simulink model "Praktikum05"  (R2023b)
settings: Solver=VariableStepAuto  StartTime=0.0  StopTime=0.01  RelTol=1e-3
model workspace (MAT data in the model file):
  CodeRate = 0.75
  M = 16
  PunctureVector = [1; 1; 0; 1; 0; 1]
  TracebackDepth = 48
  Trelli.numInputSymbols = 2
  Trelli.numOutputSymbols = 4
  Trelli.numStates = 64
  Trelli.nextStates = [0  32; 0  32; 1  33; 1  33; 2  34; 2  34; 3  35; 3  35; 4  36; 4  36; 5  37; 5  37; 6  38; 6  38; 7  39; 7  39; 8  40; 8  40; 9  41; 9  41; 10  42; 10  42; 11  43; 11  43; 12  44; 12  44; 13  45; 13  45; 14  46; 14  46; 15  47; 15  47; 16  48; 16  48; 17  49; 17  49; 18  50; 18  50; 19  51; 19  51; 20  52; 20  52; 21  53; 21  53; 22  54; 22  54; 23  55; 23  55; 24  56; 24  56; 25  57; 25  57; 26  58; 26  58; 27  59; 27  59; 28  60; 28  60; 29  61; 29  61; 30  62; 30  62; 31  63; 31  63]
  Trelli.outputs = [0  3; 3  0; 1  2; 2  1; 0  3; 3  0; 1  2; 2  1; 3  0; 0  3; 2  1; 1  2; 3  0; 0  3; 2  1; 1  2; 3  0; 0  3; 2  1; 1  2; 3  0; 0  3; 2  1; 1  2; 0  3; 3  0; 1  2; 2  1; 0  3; 3  0; 1  2; 2  1; 2  1; 1  2; 3  0; 0  3; 2  1; 1  2; 3  0; 0  3; 1  2; 2  1; 0  3; 3  0; 1  2; 2  1; 0  3; 3  0; 1  2; 2  1; 0  3; 3  0; 1  2; 2  1; 0  3; 3  0; 2  1; 1  2; 3  0; 0  3; 2  1; 1  2; 3  0; 0  3]
  Ts = 5e-08
undefined symbols (not defined in the file or in its folder): doppler, magnitude
libraries: commchan3 x2, commrflib2 x2, commsink2 x2, commdigbbndam3 x2, dspquant2 x2, commcnvcod2 x2, dspxfrm3 x1, dspstat3 x1, dspindex x1, dspmathops x1
settings Model: Creator=suttarar@hu-berlin.de  LastModifiedBy=suttarar@hu-berlin.de

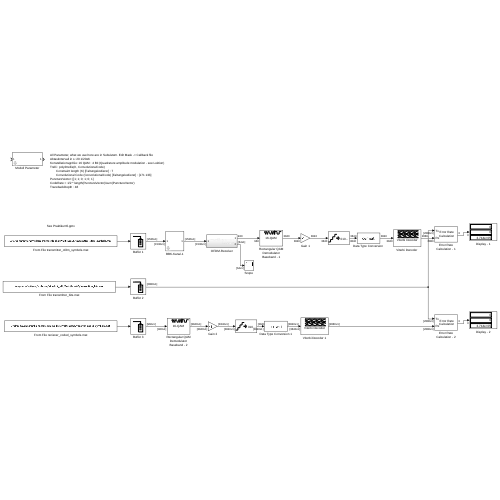
[thumbnail: Simulink's stored preview of the top-level diagram]
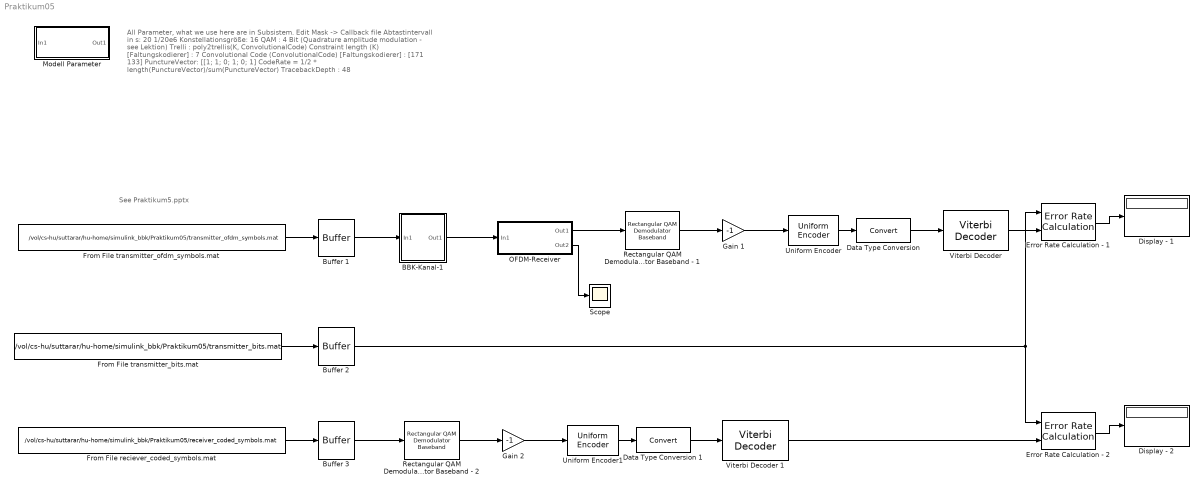
== system Praktikum05 ==
  note: See Praktikum5.pptx
  note: All Parameter, what we use here are in Subsistem. Edit Mask -> Callback file
      | Abtastintervall in s: 20 1/20e6
      | Konstellationsgröße: 16 QAM : 4 Bit (Quadrature amplitude modulation - see Lektion)
      | Trelli : poly2trellis(K, ConvolutionalCode)
      | Constraint length (K) [Faltungskodierer] : 7
      | Convolutional Code (ConvolutionalCode) [Faltungskodierer] : [171 133]
      | PunctureVector: [[1; 1; 0; 1; 0; 1]
      | CodeRate = 1/2 * length(PunctureVector)/sum(PunctureVector)
      | TracebackDepth : 48
  BBK-Kanal-1 : Subsystem  mask{MaxDoppler=0, PathDelays=0, PathGains=0, EnableMultipath=0, PathLoss=0, FrequencyOffset=0, PhaseOffset=0, SNR=15}
      mask prompts: MaxDoppler "Dopplerverschiebung"; PathDelays "Pfadverzoergerungen"; PathGains "Pfadverstaerkungen"; EnableMultipath "SwitchBlock"; PathLoss "Pfadverlust"; FrequencyOffset "Frequenzverschiebung"; PhaseOffset "Phasenverschiebung"; SNR "AWG-Rauschen"
  Buffer 1 : Buffer  N=64*24  OutputFrames=off
  Buffer 2 : Buffer  N=48*20*log2(M)*CodeRate  OutputFrames=off
  Buffer 3 : Buffer  N=48*20  OutputFrames=off
  "Data Type Conversion " : DataTypeConversion  SaturateOnIntegerOverflow=off  RndMeth=Floor
  Data Type Conversion 1 : DataTypeConversion  SaturateOnIntegerOverflow=off  RndMeth=Floor
  Display - 1 : Display
  Display - 2 : Display
  Error Rate Calculation - 1 : commsink2/Error Rate Calculation  N=TracebackDepth  st_delay=48*20*log2(M)*CodeRate  cp_mode=Entire frame  subframe=[]  PMode=Port  WsName=ErrorVec  RsMode2=off  stop=off  numErr=100  maxBits=1e6
  Error Rate Calculation - 2 : commsink2/Error Rate Calculation  N=TracebackDepth  st_delay=48*20*log2(M)*CodeRate  cp_mode=Entire frame  subframe=[]  PMode=Port  WsName=ErrorVec  RsMode2=off  stop=off  numErr=100  maxBits=1e6
  From File reciever_coded_symbols.mat : FromFile  FileName=/vol/cs-hu/suttarar/hu-home/simulink_bbk/Praktikum05/receiver_coded_symbols.mat  SampleTime=Ts/(48*20)*64*24
  From File transmitter_bits.mat : FromFile  FileName=/vol/cs-hu/suttarar/hu-home/simulink_bbk/Praktikum05/transmitter_bits.mat  SampleTime=Ts/(48*20*log2(M)*CodeRate)*64*24
  From File transmitter_ofdm_symbols.mat : FromFile  FileName=/vol/cs-hu/suttarar/hu-home/simulink_bbk/Praktikum05/transmitter_ofdm_symbols.mat  SampleTime=Ts
  Gain 1 : Gain  Gain=-1
  Gain 2 : Gain  Gain=-1
  Modell Parameter : Subsystem  mask{Ts=1/20e6, M=16, Trelli=poly2trellis(7, [171 133]), PunctureVector=[1; 1; 0; 1; 0; 1], CodeRate=0.75, TracebackDepth=48}
      mask prompts: Ts "Abtastintervall in s"; M "Konstellationsgröße"
  OFDM-Receiver : Subsystem
  Rectangular QAM Demodulator Baseband - 1 : commdigbbndam3/Rectangular QAM Demodulator Baseband  M=M  OutType=Bit  DecType=Approximate log-likelihood ratio  VarSource=Dialog  Variance=1  Dec=Gray  Mapping=[0:15]  PowType=Average Power  MinDist=2  AvgPow=1  PeakPow=1  Ph=0  outDtype1=Inherit via internal rule  outDtype2=Inherit via internal rule  derotateFactorWordLen=16  derotateFactorDataTypeStr=Inherit: Same word length as input  derotateFactorLastDataTypeStr=Inherit: Same word length as input  denormFactorWordLen=16  denormFactorDataTypeStr=Inherit: Same word length as input  denormFactorLastDataTypeStr=Inherit: Same word length as input  prodOutWordLen=32  prodOutOverflowMode=Wrap  prodOutRoundingMode=Floor  prodOutOvFlMode=off  prodOutOvFlModeLastStrValue=off  sumWordLen=32
  Rectangular QAM Demodulator Baseband - 2 : commdigbbndam3/Rectangular QAM Demodulator Baseband  M=M  OutType=Bit  DecType=Approximate log-likelihood ratio  VarSource=Dialog  Variance=1  Dec=Gray  Mapping=[0:15]  PowType=Average Power  MinDist=2  AvgPow=1  PeakPow=1  Ph=0  outDtype1=Inherit via internal rule  outDtype2=Inherit via internal rule  derotateFactorWordLen=16  derotateFactorDataTypeStr=Inherit: Same word length as input  derotateFactorLastDataTypeStr=Inherit: Same word length as input  denormFactorWordLen=16  denormFactorDataTypeStr=Inherit: Same word length as input  denormFactorLastDataTypeStr=Inherit: Same word length as input  prodOutWordLen=32  prodOutOverflowMode=Wrap  prodOutRoundingMode=Floor  prodOutOvFlMode=off  prodOutOvFlModeLastStrValue=off  sumWordLen=32
  "Scope " : Scope
  Uniform Encoder : dspquant2/Uniform Encoder  peak=1  bits=4  otype=Unsigned integer
  Uniform Encoder1 : dspquant2/Uniform Encoder  peak=1  bits=4  otype=Unsigned integer
  "Viterbi Decoder " : commcnvcod2/Viterbi Decoder  trellis=Trelli  isPunctured=on  punctureVector=PunctureVector  erasures=off  dectype=Soft decision  nsdecb=4  runSigValErrCheck=off  tbdepth=TracebackDepth  opmode=Continuous  reset=off  delayedResetAction=off  smWordLength=16  outDataType=double
  Viterbi Decoder 1 : commcnvcod2/Viterbi Decoder  trellis=Trelli  isPunctured=on  punctureVector=PunctureVector  erasures=off  dectype=Soft decision  nsdecb=4  runSigValErrCheck=off  tbdepth=TracebackDepth  opmode=Continuous  reset=off  delayedResetAction=off  smWordLength=16  outDataType=double
  wires:
  Buffer 1/1 -> BBK-Kanal-1/1(In1)
  BBK-Kanal-1/1(Out1) -> OFDM-Receiver/1(In1)
  "Data Type Conversion "/1 -> "Viterbi Decoder "/1
  "Viterbi Decoder "/1 -> Error Rate Calculation - 1/2
  Error Rate Calculation - 1/1 -> Display - 1/1
  Uniform Encoder/1 -> "Data Type Conversion "/1
  Rectangular QAM Demodulator Baseband - 1/1 -> Gain 1/1
  Gain 1/1 -> Uniform Encoder/1
  OFDM-Receiver/1(Out1) -> Rectangular QAM Demodulator Baseband - 1/1
  From File transmitter_bits.mat/1 -> Buffer 2/1
  OFDM-Receiver/2(Out2) -> "Scope "/1
  From File transmitter_ofdm_symbols.mat/1 -> Buffer 1/1
  Error Rate Calculation - 2/1 -> Display - 2/1
  From File reciever_coded_symbols.mat/1 -> Buffer 3/1
  Buffer 3/1 -> Rectangular QAM Demodulator Baseband - 2/1
  Data Type Conversion 1/1 -> Viterbi Decoder 1/1
  Gain 2/1 -> Uniform Encoder1/1
  Rectangular QAM Demodulator Baseband - 2/1 -> Gain 2/1
  Uniform Encoder1/1 -> Data Type Conversion 1/1
  Viterbi Decoder 1/1 -> Error Rate Calculation - 2/2
  Buffer 2/1 -> Error Rate Calculation - 2/1, Error Rate Calculation - 1/1

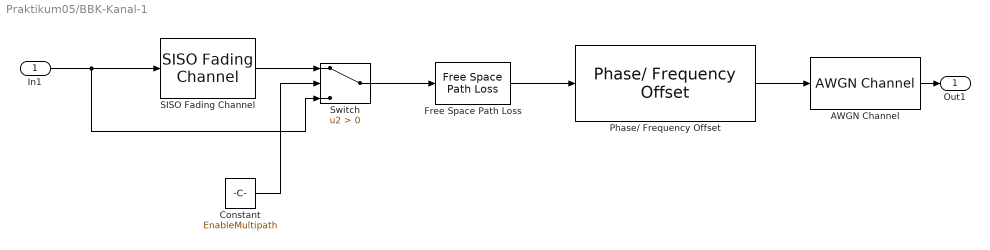
== system Praktikum05/BBK-Kanal-1 ==
  In1 : Inport
  AWGN Channel : commchan3/AWGN Channel  LegacyMode=off  NoiseMethod="Signal to noise ratio  (SNR)"  noiseMode="Signal to noise ratio  (SNR)"  EbNo=10  EsNo=10  SNR=SNR  BitsPerSymbol=1  SignalPower=1  SamplesPerSymbol=1  SymbolPeriod=1  VarianceSource=Parameter  Variance=1  RandomStream=Global stream  Seed=67  SimulateUsing=Code generation
  Constant : Constant  Value=EnableMultipath
  Free Space Path Loss : commrflib2/Free Space Path Loss  mode=Decibels  dB=PathLoss  d=0.100  fc=1920
  Phase/ Frequency Offset : commrflib2/Phase// Frequency Offset  phaseOffset=PhaseOffset  freqPort=off  freqOffset=FrequencyOffset
      settings: LibrarySourceBlock=|
      | commrfcorlib/Phase//
      | Frequency
      | Offset
  SISO Fading Channel : commchan3/SISO Fading Channel  InheritSampleRate=on  SampleRate=1  PathDelays=PathDelays  AveragePathGains=PathGains  NormalizePathGains=on  FadingDistribution=Rayleigh  KFactor=3  DirectPathDopplerShift=0  DirectPathInitialPhase=0  MaximumDopplerShift=MaxDoppler  DopplerSpectrum=doppler('Jakes')  RandomStream=mt19937ar with seed  Seed=73  PathGainsOutputPort=off  ChannelFilterDelayOutputPort=off  SimulateUsing=Interpreted execution  Visualization=Off  PathsForDopplerDisplay=1  SamplesToDisplay=25%
  Switch : Switch  Criteria=u2 > Threshold  SaturateOnIntegerOverflow=off  InputSameDT=off
  Out1 : Outport
  wires:
  Phase/ Frequency Offset/1 -> AWGN Channel/1
  Free Space Path Loss/1 -> Phase/ Frequency Offset/1
  AWGN Channel/1 -> Out1/1
  Switch/1 -> Free Space Path Loss/1
  SISO Fading Channel/1 -> Switch/1
  In1/1 -> Switch/3, SISO Fading Channel/1
  Constant/1 -> Switch/2

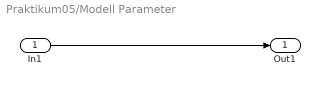
== system Praktikum05/Modell Parameter ==
  In1 : Inport
  Out1 : Outport
  wires:
  In1/1 -> Out1/1

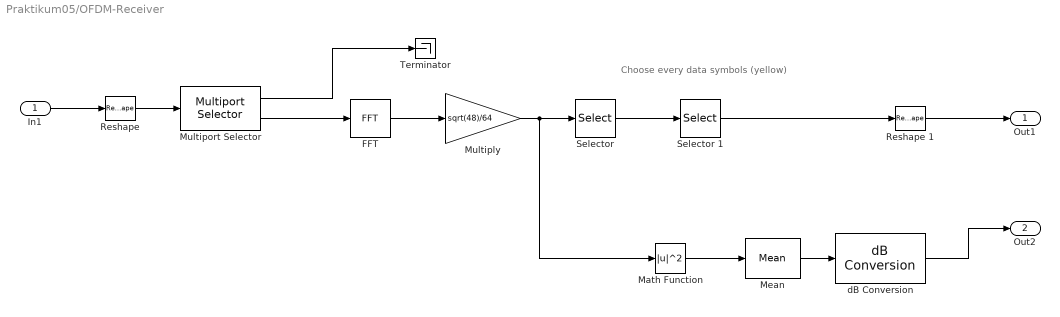
== system Praktikum05/OFDM-Receiver ==
  note: Choose every data symbols (yellow)
  In1 : Inport
  "FFT " : dspxfrm3/FFT  FFTImplementation=Auto  CompMethod=Table lookup  TableOpt=NEW  TableOptActive=Speed  BitRevOrder=off  Normalize=off  InheritFFTLength=on  FFTLength=64  WrapInput=on  roundingMode=Floor  overflowMode=off  firstCoeffDataTypeStr=Inherit: Same word length as input  firstCoeffLastDataTypeStr=Inherit: Same word length as input  outputMin=[]  outputMax=[]
  "Math Function " : Math  Operator=magnitude^2
  "Mean " : dspstat3/Mean  run=off  InputProcessing=Columns as channels (frame based)  reset_popup=None  directionMode=Each row  dimension=1  roiEnable=off  roiType=Rectangles  roiPortion=Entire ROI  roiOutput=Individual statistics for each ROI  roiFlag=off  roundingMode=Floor  overflowMode=off  outputDataTypeStr=Inherit: Same as accumulator  outputMin=[]  outputMax=[]  outputLastDataTypeStr=Inherit: Same as accumulator
  "Multiply " : Gain  Gain=sqrt(48)/64
  "Multiport Selector " : dspindex/Multiport Selector  rowsOrCols=Columns  idxCellArray={[1:4], [5:24]}  idxErrMode=Clip Index
  "Reshape " : Reshape  OutputDimensionality=Customize  OutputDimensions=[64,24]
  Reshape 1 : Reshape  OutputDimensions=[64,24]
  "Selector " : Selector  NumberOfDimensions=2  InputPortWidth=3  IndexOptions=Index vector (dialog),Select all  Indices=[39:64 1:38],1  OutputSizes=1,1
  Selector 1 : Selector  NumberOfDimensions=2  InputPortWidth=3  IndexOptions=Index vector (dialog),Select all  Indices=[1:5 7:19 21:26 28:33 35:47 49:53],1  OutputSizes=1,1
  "Terminator " : Terminator
  "dB Conversion " : dspmathops/dB Conversion  dBtype=dB  intype=Power  R=1  fuzz=off
      settings: LibrarySourceBlock=commutil2/dB Conversion
  Out1 : Outport
  Out2 : Outport  Port=2
  wires:
  "Mean "/1 -> "dB Conversion "/1
  "Math Function "/1 -> "Mean "/1
  "FFT "/1 -> "Multiply "/1
  In1/1 -> "Reshape "/1
  "Selector "/1 -> Selector 1/1
  "Reshape "/1 -> "Multiport Selector "/1
  "Multiport Selector "/2 -> "FFT "/1
  "Multiport Selector "/1 -> "Terminator "/1
  "dB Conversion "/1 -> Out2/1
  Selector 1/1 -> Reshape 1/1
  Reshape 1/1 -> Out1/1
  "Multiply "/1 -> "Math Function "/1, "Selector "/1
